simulink model "NOx_integrated_SIgnal_Builder"  (R2019a)
settings: Solver=FixedStepDiscrete  StartTime=0.0  StopTime=1500  FixedStep=0.1  RelTol=1e-3
undefined symbols (not defined in the file or in its folder): sigbuilder_block
settings Model: Creator=Kore  LastModifiedBy=admin
settings OptimizationCC: DefaultParameterBehavior=Inlined  EnhancedBackFolding=on  PassReuseOutputArgsAs=Individual arguments  OptimizeBlockOrder=speed  DifferentSizesBufferReuse=on  OptimizationCustomize=off
settings DebuggingCC: ParameterTunabilityLossMsg=error
settings SFSimCC: MATLABDynamicMemAlloc=off
settings RTWCC: SystemTargetFile=ert.tlc  GenCodeOnly=on  TemplateMakefile=ert_default_tmf  GenerateReport=on  IncludeHyperlinkInReport=on  LaunchReport=on  GenerateTraceInfo=on  GenerateTraceReport=on  GenerateTraceReportSl=on  GenerateTraceReportSf=on  GenerateTraceReportEml=on
settings CodeAppCC: ForceParamTrailComments=on  IgnoreCustomStorageClasses=off  OperatorAnnotations=on  SimulinkDataObjDesc=on  SFDataObjDesc=on  InsertBlockDesc=on
settings ERTTargetCC: TargetLangStandard=C99 (ISO)  GenerateSampleERTMain=on  InlinedParameterPlacement=NonHierarchical  ERTCustomFileTemplate=example_file_process.tlc
settings ConfigComp: CovEnable=on  RecordCoverage=on  CovMetricSettings=dcmwe  CovModelRefEnable=on

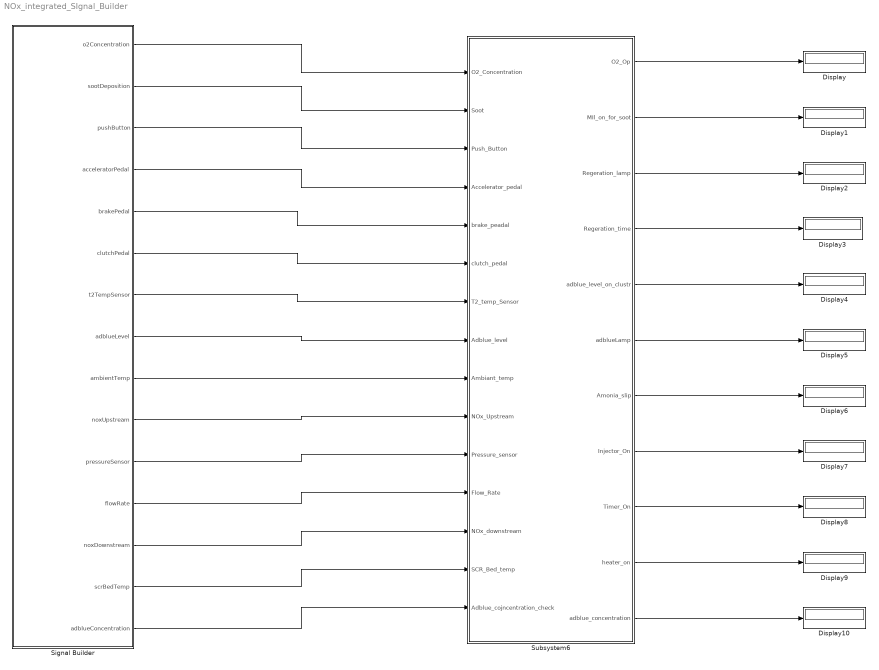
== system NOx_integrated_SIgnal_Builder ==
  Display{,1..10} (11 alike) : Display
  Signal Builder : Subsystem  Tag=STV Subsys  LoadFcn=sigbuilder_block('load');  StartFcn=sigbuilder_block('start');  StopFcn=sigbuilder_block('stop');  ClipboardFcn=sigbuilder_block('clipboard');  mask(Sigbuilder block){tuvar=[0:10]}
      mask help: Simulink:masks:SigbuilderBlock_MD
      mask init:
      | if ~strcmp(get_param(bdroot(gcbh),'SimulationStatus'),'stopped') tuvar = sigbuilder_block('maskInit'); end
      settings: CopyFcn=sigbuilder_block('copy');  DeleteFcn=sigbuilder_block('delete');  ModelCloseFcn=sigbuilder_block('modelClose');  PreSaveFcn=sigbuilder_block('preSave');  PauseFcn=sigbuilder_block('pause');  ContinueFcn=sigbuilder_block('continue');  NameChangeFcn=sigbuilder_block('namechange');  OpenFcn=sigbuilder_block('open',[437.6 30.75 550.4 481.5 ]);  CloseFcn=sigbuilder_block('close');
      mask Display: plot(0, 0, 100, 100,[2, 2, 32, 32, 2], [68, 8, 8, 68, 68],[32, 2], [38, 38], [32, 19, 2],[53, 60, 44], [32, 17, 17, 2],[16, 16, 31, 31]);txt = getActiveGroup(gcbh);text(2, 100, txt,'verticalAlignment', 'top');
  Subsystem6 : Subsystem
  wires:
  Subsystem6/2(MIl_on_for_soot) -> Display1/1
  Subsystem6/8(Injector_On) -> Display7/1
  Subsystem6/11(adblue_concentration) -> Display10/1
  Subsystem6/9(Timer_On) -> Display8/1
  Subsystem6/5(adblue_level_on_clustr) -> Display4/1
  Subsystem6/1(O2_Op) -> Display/1
  Subsystem6/10(heater_on) -> Display9/1
  Subsystem6/7(Amonia_slip) -> Display6/1
  Subsystem6/3(Regeration_lamp) -> Display2/1
  Subsystem6/4(Regeration_time) -> Display3/1
  Subsystem6/6(adblueLamp) -> Display5/1
  Signal Builder/1(o2Concentration) -> Subsystem6/1(O2_Concentration)
  Signal Builder/2(sootDeposition) -> Subsystem6/2(Soot)
  Signal Builder/3(pushButton) -> Subsystem6/3(Push_Button)
  Signal Builder/4(acceleratorPedal) -> Subsystem6/4(Accelerator_pedal)
  Signal Builder/5(brakePedal) -> Subsystem6/5(brake_peadal)
  Signal Builder/6(clutchPedal) -> Subsystem6/6(clutch_pedal)
  Signal Builder/7(t2TempSensor) -> Subsystem6/7(T2_temp_Sensor)
  Signal Builder/8(adblueLevel) -> Subsystem6/8(Adblue_level)
  Signal Builder/9(ambientTemp) -> Subsystem6/9(Ambiant_temp)
  Signal Builder/10(noxUpstream) -> Subsystem6/10(NOx_Upstream)
  Signal Builder/11(pressureSensor) -> Subsystem6/11(Pressure_sensor)
  Signal Builder/12(flowRate) -> Subsystem6/12(Flow_Rate)
  Signal Builder/13(noxDownstream) -> Subsystem6/13(NOx_downstream)
  Signal Builder/14(scrBedTemp) -> Subsystem6/14(SCR_Bed_temp)
  Signal Builder/15(adblueConcentration) -> Subsystem6/15(Adblue_cojncentration_check)

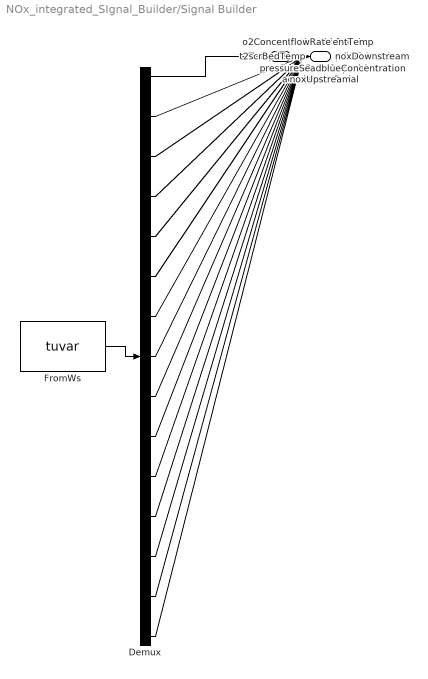
== system NOx_integrated_SIgnal_Builder/Signal Builder ==
  Demux : Demux  Tag=STV Demux  Outputs=15
  FromWs : FromWorkspace  Tag=STV FromWs  VariableName=tuvar  SampleTime=0
      SigBuilderData=|
      | common.afterFinalStr = 'Extrapolate'
      | common.sampleTime = 0
      | dataSet.timeRange = [0.1 77.4]
      | dataSet.name = 'Sheet1'
      | sbobj.Name = 'Signal Builder'
      | sbobj.Groups.Name = 'Sheet1'
      | sbobj.Groups.Signals(1).Name = 'o2Concentration'
      | sbobj.Groups.Signals(1).XData = [0.1 0.2 0.3 0.4 0.5 0.6 0.7 0.8 0.9 1 1.1 1.2 ... (774 elements, 1x774)]
      | sbobj.Groups.Signals(1).YData = [6.5 7 7.5 8 8.5 9 9.5 10 10.5 11 11.5 12 ... (774 elements, 1x774)]
      | sbobj.Groups.Signals(2).Name = 'sootDeposition'
      | sbobj.Groups.Signals(2).XData = [0.1 0.2 0.3 0.4 0.5 0.6 0.7 0.8 0.9 1 1.1 1.2 ... (774 elements, 1x774)]
      | sbobj.Groups.Signals(2).YData = [0.01 0.02 0.03 0.04 0.05 0.06 0.07 0.08 0.09 0.1 0.11 0.12 ... (774 elements, 1x774)]
      | sbobj.Groups.Signals(3).Name = 'pushButton'
      | sbobj.Groups.Signals(3).XData = [0.1 0.2 0.3 0.4 0.5 0.6 0.7 0.8 0.9 1 1.1 1.2 ... (774 elements, 1x774)]
      | sbobj.Groups.Signals(3).YData = [1 1 0 0 0 0 0 0 0 0 0 0 0 0 0 0 1 1 1 1 1 1 1 1 1 1 1 1 1 1 1 1 1 1 1 1 1 1 1 1 1 1 1 1 1 1 1 1 1 1 1 1 1 1 1 1 1 1 1 1 1 1 1 1 1 1 1 1 1 1 1 1 1 1 1 1 1 1 1 1 1 1 1 1 1 1 1 1 1 1 0 0 0 0 0 0 0 0 0 0 0 0 0 0 0 0 0 0 0 0 0 0 0 1 1 1 1 1 1 1 1 1 1 1 1 1 1 1 1 1 1 1 1 1 1 1 1 1 1 1 0 1 1 1 1 1 1 1 1 1 1 1 1 1 1 1 1 1 1 1 1 1 1 1 1 1 1 1 1 1 1 1 1 1 1 1 1 1 1 1 1 1 1 1 1 1 1 1 1 1 1 1 0 0 0 0 0 0 0 0 0 0 0 0 0 0 0 0 0 0 0 0 0 0 0 0 0 0 0 0 0 0 0 0 1 1 1 1 1 1 1 1 1 1 1 1 1 1 1 1 1 1 1 1 1 1 1 1 1 1 1 1 1 1 1 1 1 1 1 1 1 1 1 1 1 1 1 1 1 1 1 1 1 1 1 1 1 1 1 1 1 1 1 1 1 1 1 1 1 1 1 1 1 1 1 1 1 1 1 1 1 0 0 0 0 0 0 0 0 0 0 0 0 0 0 0 0 0 0 0 0 0 0 0 0 0 1 1 1 1 1 1 1 1 1 1 1 1 1 1 1 1 1 1 1 1 1 1 1 1 1 1 1 1 1 1 1 1 1 1 1 1 1 1 1 1 1 1 1 1 1 1 1 1 1 1 1 1 1 1 1 1 1 1 1 1 1 1 1 1 1 1 1 1 1 1 1 1 1 1 1 1 1 1 1 1 1 1 1 1 1 1 1 1 1 1 1 1 1 1 1 1 1 1 1 1 1 1 1 1 1 1 1 1 1 1 1 1 1 1 1 1 1 1 1 1 1 1 1 1 1 1 1 1 1 1 1 1 1 1 1 1 1 1 1 1 1 1 1 1 1 1 1 1 1 1 1 1 1 1 1 1 1 1 1 1 1 1 1 1 1 1 1 1 1 1 1 1 1 1 1 1 1 1 1 1 1 1 1 1 1 1 1 1 1 1 1 1 1 1 1 1 1 1 1 1 1 1 1 1 1 1 1 1 1 1 1 1 1 1 1 1 1 1 1 1 1 1 1 1 1 1 1 1 1 1 1 1 1 1 1 1 1 1 1 1 1 1 1 1 1 1 1 1 1 1 1 1 1 1 1 1 1 1 1 1 1 1 1 1 1 1 1 1 1 1 1 1 1 1 1 1 1 1 1 1 1 1 1 1 1 1 1 1 1 1 1 1 1 1 1 1 1 1 1 1 1 1 1 1 1 1 1 1 1 1 1 1 1 1 1 1 1 1 1 1 1 1 1 1 1 1 1 1 1 1 1 1 1 1 1 1 1 1 1 1 1 1 1 1 1 1 1 1 1 1 1 1 1 1 1 1 1 1 1 1 1 1 1 1 1 1 1 1 1 1 1 1 1 1 1 1 1 1 1 1 1 1 1 1 1 1 1 1 1 1 1 1 1 1 1 1 1 1 1 1 1 1 1 1 1 1 1 1 1 1 1 1 1 1 1 1 1 1 1 1 0 0 0 0 0 0 0 0 1 1 1 1 1 1 1 1 1 0 0 0 0 0 0 0 0 0 1 1]
      | sbobj.Groups.Signals(4).Name = 'acceleratorPedal'
      | sbobj.Groups.Signals(4).XData = [0.1 0.2 0.3 0.4 0.5 0.6 0.7 0.8 0.9 1 1.1 1.2 ... (774 elements, 1x774)]
      | sbobj.Groups.Signals(4).YData = [0 0 0 0 0 0 0 0 0 0 0 0 0 0 0 0 0 0 0 0 0 0 0 0 0 0 0 0 1 1 1 1 1 1 1 1 1 1 1 1 1 1 1 1 1 1 1 1 1 1 1 1 1 0 0 0 0 0 0 0 0 0 0 0 0 0 0 0 0 0 0 0 0 0 0 0 0 0 0 0 0 0 0 0 0 0 0 0 0 0 0 0 0 0 0 0 0 0 0 0 0 0 0 0 0 0 0 0 0 0 0 0 0 0 0 0 0 0 0 0 0 0 0 0 0 0 0 0 0 0 0 0 0 0 0 0 0 0 0 0 0 0 0 0 0 1 0 0 0 0 0 0 1 0 0 0 0 0 1 1 0 0 0 0 0 1 0 0 0 0 0 0 0 0 0 0 0 1 0 0 0 0 0 1 0 0 1 0 0 0 0 0 0 0 0 0 0 0 0 0 0 0 0 0 0 0 0 0 0 0 0 0 0 0 0 0 0 0 0 0 0 0 0 0 0 0 0 0 0 0 0 0 0 0 0 0 0 0 0 0 0 0 0 0 0 0 0 0 0 0 0 0 0 0 0 0 0 0 0 0 0 0 0 0 0 0 0 0 0 0 0 0 0 0 0 0 0 0 0 0 0 0 0 0 0 0 0 0 0 0 0 0 0 0 0 0 0 0 0 0 0 1 1 1 1 1 1 1 1 1 1 1 1 1 1 1 1 1 1 1 1 1 1 1 1 1 0 0 0 0 0 0 0 0 0 0 0 0 0 0 0 0 0 0 0 0 0 0 0 0 0 0 0 0 0 0 0 0 0 0 0 0 0 0 0 0 0 0 0 0 0 0 0 0 0 0 0 0 0 0 0 0 0 0 0 0 0 0 0 0 0 0 0 0 0 0 0 0 0 0 0 0 0 0 0 0 0 0 0 0 0 0 0 0 0 0 0 0 0 0 0 0 0 0 0 0 0 0 0 0 0 0 0 0 0 0 0 0 0 0 0 0 0 0 0 0 0 0 0 0 0 0 0 0 0 0 0 0 0 0 0 0 0 0 0 0 0 0 0 0 0 0 0 0 0 0 0 0 0 0 0 0 0 0 0 0 0 0 0 0 0 0 0 0 0 0 0 0 0 0 0 0 0 0 0 0 0 0 0 0 0 0 0 0 0 0 0 0 0 0 0 0 0 0 0 0 0 0 0 0 0 0 0 0 0 0 0 0 0 0 0 0 0 0 0 1 0 0 0 0 0 0 1 0 0 0 0 0 1 1 0 0 0 0 0 1 0 0 0 0 0 0 0 0 0 0 0 1 0 0 0 0 0 1 0 0 1 0 0 0 0 0 0 0 0 0 0 0 0 0 0 0 0 0 0 0 0 0 0 0 0 0 0 0 0 0 0 0 0 0 0 0 0 0 0 0 0 0 0 0 0 0 0 0 0 0 0 0 0 0 0 0 0 0 0 0 0 0 0 0 0 0 0 0 0 0 0 0 0 0 0 0 0 0 0 0 0 0 0 0 0 0 0 0 0 0 0 0 0 0 0 0 0 0 0 0 0 0 0 0 0 0 0 0 0 0 0 0 0 0 0 0 0 0 0 0 0 0 0 0 0 0 0 0 0 0 0 1 1 0 1 0 0 0 1 1 1 1 1 1 1 1 0 0 0 1 1 1 1 0 0 0 0 1 1 1 0 0 0 0 1 1 1 0 0 0 0 1 1 1 0 0 0 0 0 0 0 0 1 1 1 0 0 0]
      | sbobj.Groups.Signals(5).Name = 'brakePedal'
      | sbobj.Groups.Signals(5).XData = [0.1 0.2 0.3 0.4 0.5 0.6 0.7 0.8 0.9 1 1.1 1.2 ... (774 elements, 1x774)]
      | sbobj.Groups.Signals(5).YData = [0 0 0 0 0 0 0 0 0 0 0 0 0 0 0 0 0 0 0 0 0 0 0 0 0 0 0 0 1 1 1 1 1 1 1 1 1 1 1 1 1 1 1 1 1 1 1 1 1 1 1 1 1 0 0 0 0 0 0 0 0 0 0 0 0 0 0 0 0 0 0 0 0 0 0 0 0 0 0 0 0 0 0 0 0 0 0 0 0 0 0 0 0 0 0 0 0 0 0 0 0 0 0 0 0 0 0 0 0 0 0 0 0 0 0 0 0 0 0 0 0 0 0 0 0 0 0 0 0 0 0 0 0 0 0 0 0 0 0 0 0 0 0 0 0 0 1 0 0 0 0 0 0 1 0 0 0 1 0 0 1 0 0 1 0 0 0 0 0 1 0 1 0 1 0 0 0 0 0 0 0 0 0 0 0 0 0 0 0 0 0 0 0 0 0 0 0 0 0 0 0 0 0 0 0 0 0 0 0 0 0 0 0 0 0 0 0 0 0 0 0 0 0 0 0 0 0 0 0 0 0 0 0 0 0 0 0 0 0 0 0 0 0 0 0 0 0 0 0 0 0 0 0 0 0 0 0 0 0 0 0 0 0 0 0 0 0 0 0 0 0 0 0 0 0 0 0 0 0 0 0 0 0 0 0 0 0 0 0 0 0 0 0 0 0 0 0 0 0 0 0 1 1 1 1 1 1 1 1 1 1 1 1 1 1 1 1 1 1 1 1 1 1 1 1 1 0 0 0 0 0 0 0 0 0 0 0 0 0 0 0 0 0 0 0 0 0 0 0 0 0 0 0 0 0 0 0 0 0 0 0 0 0 0 0 0 0 0 0 0 0 0 0 0 0 0 0 0 0 0 0 0 0 0 0 0 0 0 0 0 0 0 0 0 0 0 0 0 0 0 0 0 0 0 0 0 0 0 0 0 0 0 0 0 0 0 0 0 0 0 0 0 0 0 0 0 0 0 0 0 0 0 0 0 0 0 0 0 0 0 0 0 0 0 0 0 0 0 0 0 0 0 0 0 0 0 0 0 0 0 0 0 0 0 0 0 0 0 0 0 0 0 0 0 0 0 0 0 0 0 0 0 0 0 0 0 0 0 0 0 0 0 0 0 0 0 0 0 0 0 0 0 0 0 0 0 0 0 0 0 0 0 0 0 0 0 0 0 0 0 0 0 0 0 0 0 0 0 0 0 0 0 0 0 0 0 0 0 0 0 0 0 0 0 0 0 1 0 0 0 0 0 0 1 0 0 0 1 0 0 1 0 0 1 0 0 0 0 0 1 0 1 0 1 0 0 0 0 0 0 0 0 0 0 0 0 0 0 0 0 0 0 0 0 0 0 0 0 0 0 0 0 0 0 0 0 0 0 0 0 0 0 0 0 0 0 0 0 0 0 0 0 0 0 0 0 0 0 0 0 0 0 0 0 0 0 0 0 0 0 0 0 0 0 0 0 0 0 0 0 0 0 0 0 0 0 0 0 0 0 0 0 0 0 0 0 0 0 0 0 0 0 0 0 0 0 0 0 0 0 0 0 0 0 0 0 0 0 0 0 0 0 0 0 0 0 0 0 0 0 0 0 0 0 0 0 0 0 0 0 0 0 0 0 0 0 0 1 1 0 1 0 0 1 1 1 1 1 1 1 1 1 0 0 0 1 1 1 1 0 0 0 0 1 1 1 0 0 0 0 1 1 1 0 0 0 0 1 1 1 0 0 0 0 0 0 0 0 1 1 1 0 0 0]
      | sbobj.Groups.Signals(6).Name = 'clutchPedal'
      | sbobj.Groups.Signals(6).XData = [0.1 0.2 0.3 0.4 0.5 0.6 0.7 0.8 0.9 1 1.1 1.2 ... (774 elements, 1x774)]
      | sbobj.Groups.Signals(6).YData = [0 0 0 0 0 0 0 0 0 0 0 0 0 0 0 0 0 0 0 0 0 0 0 0 0 0 0 0 1 1 1 1 1 1 1 1 1 1 1 1 1 1 1 1 1 1 1 1 1 1 1 1 1 0 0 0 0 0 0 0 0 0 0 0 0 0 0 0 0 0 0 0 0 0 0 0 0 0 0 0 0 0 0 0 0 0 0 0 0 0 0 0 0 0 0 0 0 0 0 0 0 0 0 0 0 0 0 0 0 0 0 0 0 0 0 0 0 0 0 0 0 0 0 0 0 0 0 0 0 0 0 0 0 0 0 0 0 0 0 0 0 0 0 0 0 0 0 1 0 0 0 0 0 0 1 0 0 0 1 0 0 0 0 0 1 0 0 0 0 0 0 0 0 0 0 1 0 0 1 0 0 0 0 0 1 0 0 0 0 0 0 0 0 0 0 0 0 0 0 0 0 0 0 0 0 0 0 0 0 0 0 0 0 0 0 0 0 0 0 0 0 0 0 0 0 0 0 0 0 0 0 0 0 0 0 0 0 0 0 0 0 0 0 0 0 0 0 0 0 0 0 0 0 0 0 0 0 0 0 0 0 0 0 0 0 0 0 0 0 0 0 0 0 0 0 0 0 0 0 0 0 0 0 0 0 0 0 0 0 0 0 0 0 0 0 0 0 0 0 0 0 1 1 1 1 1 1 1 1 1 1 1 1 1 1 1 1 1 1 1 1 1 1 1 1 1 0 0 0 0 0 0 0 0 0 0 0 0 0 0 0 0 0 0 0 0 0 0 0 0 0 0 0 0 0 0 0 0 0 0 0 0 0 0 0 0 0 0 0 0 0 0 0 0 0 0 0 0 0 0 0 0 0 0 0 0 0 0 0 0 0 0 0 0 0 0 0 0 0 0 0 0 0 0 0 0 0 0 0 0 0 0 0 0 0 0 0 0 0 0 0 0 0 0 0 0 0 0 0 0 0 0 0 0 0 0 0 0 0 0 0 0 0 0 0 0 0 0 0 0 0 0 0 0 0 0 0 0 0 0 0 0 0 0 0 0 0 0 0 0 0 0 0 0 0 0 0 0 0 0 0 0 0 0 0 0 0 0 0 0 0 0 0 0 0 0 0 0 0 0 0 0 0 0 0 0 0 0 0 0 0 0 0 0 0 0 0 0 0 0 0 0 0 0 0 0 0 0 0 0 0 0 0 0 0 0 0 0 0 0 0 0 0 0 0 0 0 1 0 0 0 0 0 0 1 0 0 0 1 0 0 0 0 0 1 0 0 0 0 0 0 0 0 0 0 1 0 0 1 0 0 0 0 0 1 0 0 0 0 0 0 0 0 0 0 0 0 0 0 0 0 0 0 0 0 0 0 0 0 0 0 0 0 0 0 0 0 0 0 0 0 0 0 0 0 0 0 0 0 0 0 0 0 0 0 0 0 0 0 0 0 0 0 0 0 0 0 0 0 0 0 0 0 0 0 0 0 0 0 0 0 0 0 0 0 0 0 0 0 0 0 0 0 0 0 0 0 0 0 0 0 0 0 0 0 0 0 0 0 0 0 0 0 0 0 0 0 0 0 0 0 0 0 0 0 0 0 0 0 0 0 0 0 0 0 0 0 1 1 0 1 0 0 0 1 1 1 1 1 1 1 1 0 0 0 1 1 1 1 0 0 0 0 1 1 1 0 0 0 0 1 1 1 0 0 0 0 1 1 1 0 0 0 0 0 0 0 0 1 1 1 0 0 0]
      | sbobj.Groups.Signals(7).Name = 't2TempSensor'
      | sbobj.Groups.Signals(7).XData = [0.1 0.2 0.3 0.4 0.5 0.6 0.7 0.8 0.9 1 1.1 1.2 ... (774 elements, 1x774)]
      | sbobj.Groups.Signals(7).YData = [310 320 330 340 350 360 370 380 390 400 410 420 ... (774 elements, 1x774)]
      | sbobj.Groups.Signals(8).Name = 'adblueLevel'
      | sbobj.Groups.Signals(8).XData = [0.1 0.2 0.3 0.4 0.5 0.6 0.7 0.8 0.9 1 1.1 1.2 ... (774 elements, 1x774)]
      | sbobj.Groups.Signals(8).YData = [1 2 3 4 5 6 7 8 9 10 11 12 ... (774 elements, 1x774)]
      | sbobj.Groups.Signals(9).Name = 'ambientTemp'
      | sbobj.Groups.Signals(9).XData = [0.1 0.2 0.3 0.4 0.5 0.6 0.7 0.8 0.9 1 1.1 1.2 ... (774 elements, 1x774)]
      | sbobj.Groups.Signals(9).YData = [0 1 2 3 4 5 6 7 8 9 10 11 ... (774 elements, 1x774)]
      | sbobj.Groups.Signals(10).Name = 'noxUpstream'
      | sbobj.Groups.Signals(10).XData = [0.1 0.2 0.3 0.4 0.5 0.6 0.7 0.8 0.9 1 1.1 1.2 ... (774 elements, 1x774)]
      | sbobj.Groups.Signals(10).YData = [10 70 77.6 80.4 86.4 99.6 108 117.6 127.2 136.8 149.3 158.3 ... (774 elements, 1x774)]
      | sbobj.Groups.Signals(11).Name = 'pressureSensor'
      | sbobj.Groups.Signals(11).XData = [0.1 0.2 0.3 0.4 0.5 0.6 0.7 0.8 0.9 1 1.1 1.2 ... (774 elements, 1x774)]
      | sbobj.Groups.Signals(11).YData = [5.8 5.8 5.8 5.8 5.8 5.8 5.8 5.8 5.8 5.8 5.8 5.8 ... (774 elements, 1x774)]
      | sbobj.Groups.Signals(12).Name = 'flowRate'
      | sbobj.Groups.Signals(12).XData = [0.1 0.2 0.3 0.4 0.5 0.6 0.7 0.8 0.9 1 1.1 1.2 ... (774 elements, 1x774)]
      | sbobj.Groups.Signals(12).YData = [3 3 3 3 3 4 4 4 4 4.8 4.8 4.8 ... (774 elements, 1x774)]
      | sbobj.Groups.Signals(13).Name = 'noxDownstream'
      | sbobj.Groups.Signals(13).XData = [0.1 0.2 0.3 0.4 0.5 0.6 0.7 0.8 0.9 1 1.1 1.2 ... (774 elements, 1x774)]
      | sbobj.Groups.Signals(13).YData = [15 15 15 14 14 14 14 15 15 15 15 17 ... (774 elements, 1x774)]
      | sbobj.Groups.Signals(14).Name = 'scrBedTemp'
      | sbobj.Groups.Signals(14).XData = [0.1 0.2 0.3 0.4 0.5 0.6 0.7 0.8 0.9 1 1.1 1.2 ... (774 elements, 1x774)]
      | sbobj.Groups.Signals(14).YData = [1 10 20 30 40 50 60 70 80 90 100 110 ... (774 elements, 1x774)]
      | sbobj.Groups.Signals(15).Name = 'adblueConcentration'
      | sbobj.Groups.Signals(15).XData = [0.1 0.2 0.3 0.4 0.5 0.6 0.7 0.8 0.9 1 1.1 1.2 ... (774 elements, 1x774)]
      | sbobj.Groups.Signals(15).YData = [31.5 31.6 31.7 31.8 31.9 32 32.1 32.2 32.3 32.4 32.5 32.6 ... (774 elements, 1x774)]
      | sbobj.Groups.TimeRange = [0.1 73.9]
  o2Concentration : Outport  Tag=STV Outport
  sootDeposition : Outport  Tag=STV Outport  Port=2
  pushButton : Outport  Tag=STV Outport  Port=3
  acceleratorPedal : Outport  Tag=STV Outport  Port=4
  brakePedal : Outport  Tag=STV Outport  Port=5
  clutchPedal : Outport  Tag=STV Outport  Port=6
  t2TempSensor : Outport  Tag=STV Outport  Port=7
  adblueLevel : Outport  Tag=STV Outport  Port=8
  ambientTemp : Outport  Tag=STV Outport  Port=9
  noxUpstream : Outport  Tag=STV Outport  Port=10
  pressureSensor : Outport  Tag=STV Outport  Port=11
  flowRate : Outport  Tag=STV Outport  Port=12
  noxDownstream : Outport  Tag=STV Outport  Port=13
  scrBedTemp : Outport  Tag=STV Outport  Port=14
  adblueConcentration : Outport  Tag=STV Outport  Port=15
  wires:
  Demux/1 -> o2Concentration/1
  FromWs/1 -> Demux/1
  Demux/2 -> sootDeposition/1
  Demux/3 -> pushButton/1
  Demux/4 -> acceleratorPedal/1
  Demux/5 -> brakePedal/1
  Demux/6 -> clutchPedal/1
  Demux/7 -> t2TempSensor/1
  Demux/8 -> adblueLevel/1
  Demux/9 -> ambientTemp/1
  Demux/10 -> noxUpstream/1
  Demux/11 -> pressureSensor/1
  Demux/12 -> flowRate/1
  Demux/13 -> noxDownstream/1
  Demux/14 -> scrBedTemp/1
  Demux/15 -> adblueConcentration/1

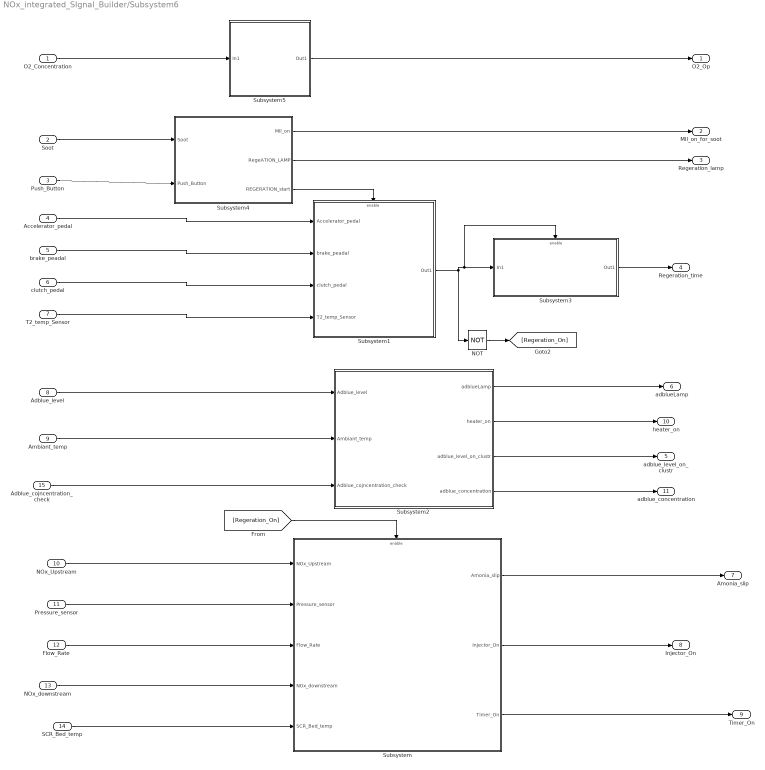
== system NOx_integrated_SIgnal_Builder/Subsystem6 ==
  O2_Concentration : Inport
  Soot : Inport  Port=2
  Push_Button : Inport  Port=3
  Accelerator_pedal : Inport  Port=4
  brake_peadal : Inport  Port=5
  clutch_pedal : Inport  Port=6
  T2_temp_Sensor : Inport  Port=7
  Adblue_level : Inport  Port=8
  Ambiant_temp : Inport  Port=9
  NOx_Upstream : Inport  Port=10
  Pressure_sensor : Inport  Port=11
  Flow_Rate : Inport  Port=12
  NOx_downstream : Inport  Port=13
  SCR_Bed_temp : Inport  Port=14
  Adblue_cojncentration_check : Inport  Port=15
  NOT : Logic  Operator=NOT  IconShape=distinctive  AllPortsSameDT=off  OutDataTypeStr=boolean
  Subsystem : Subsystem
  Subsystem1 : Subsystem
  Subsystem2 : Subsystem
  Subsystem3 : Subsystem
  Subsystem4 : Subsystem
  Subsystem5 : Subsystem
  O2_Op : Outport
  MIl_on_for_soot : Outport  Port=2
  Regeration_lamp : Outport  Port=3
  Regeration_time : Outport  Port=4
  adblue_level_on_clustr : Outport  Port=5
  adblueLamp : Outport  Port=6
  Amonia_slip : Outport  Port=7
  Injector_On : Outport  Port=8
  Timer_On : Outport  Port=9
  heater_on : Outport  Port=10
  adblue_concentration : Outport  Port=11
  wires:
  T2_temp_Sensor/1 -> Subsystem1/4(T2_temp_Sensor)
  NOT/1 -> [Regeration_On]
  Subsystem/3(Timer_On) -> Timer_On/1
  Subsystem1/1(Out1) -> Subsystem3/Enable, Subsystem3/1(In1), NOT/1
  Push_Button/1 -> Subsystem4/2(Push_Button)
  Subsystem4/3(REGERATION_start) -> Subsystem1/Enable
  Subsystem/1(Amonia_slip) -> Amonia_slip/1
  NOx_Upstream/1 -> Subsystem/1(NOx_Upstream)
  Subsystem5/1(Out1) -> O2_Op/1
  Subsystem4/2(RegeATION_LAMP) -> Regeration_lamp/1
  [Regeration_On] -> Subsystem/Enable
  Adblue_level/1 -> Subsystem2/1(Adblue_level)
  O2_Concentration/1 -> Subsystem5/1(In1)
  clutch_pedal/1 -> Subsystem1/3(clutch_pedal)
  Accelerator_pedal/1 -> Subsystem1/1(Accelerator_pedal)
  Flow_Rate/1 -> Subsystem/3(Flow_Rate)
  Soot/1 -> Subsystem4/1(Soot)
  Pressure_sensor/1 -> Subsystem/2(Pressure_sensor)
  Subsystem/2(Injector_On) -> Injector_On/1
  NOx_downstream/1 -> Subsystem/4(NOx_downstream)
  SCR_Bed_temp/1 -> Subsystem/5(SCR_Bed_temp)
  Subsystem4/1(MIl_on) -> MIl_on_for_soot/1
  brake_peadal/1 -> Subsystem1/2("brake_peadal ")
  Ambiant_temp/1 -> Subsystem2/2(Ambiant_temp)
  Subsystem2/1(adblueLamp) -> adblueLamp/1
  Subsystem2/3(adblue_level_on_clustr) -> adblue_level_on_clustr/1
  Subsystem2/2(heater_on) -> heater_on/1
  Adblue_cojncentration_check/1 -> Subsystem2/3(Adblue_cojncentration_check)
  Subsystem2/4(adblue_concentration) -> adblue_concentration/1
  Subsystem3/1(Out1) -> Regeration_time/1

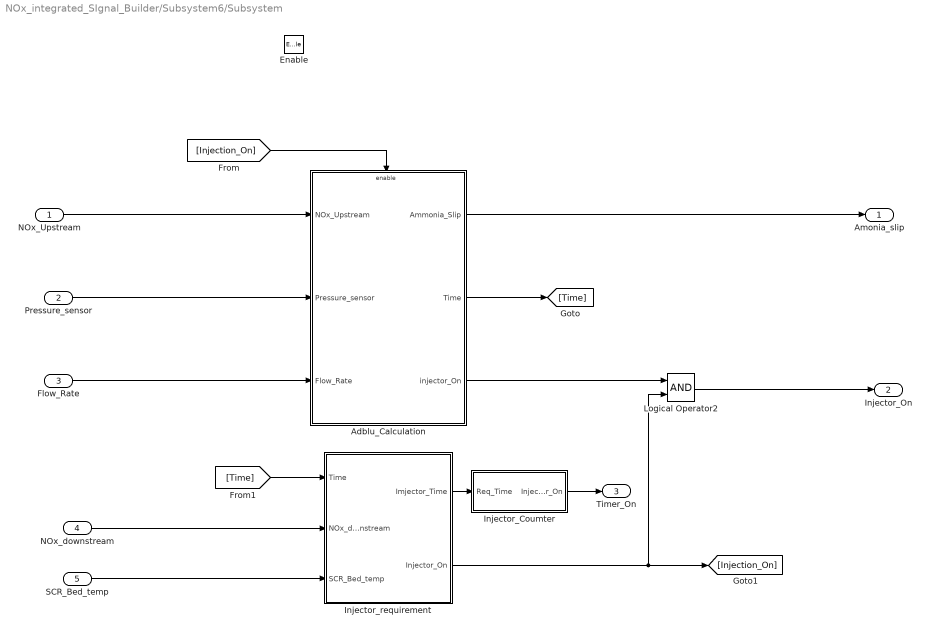
== system NOx_integrated_SIgnal_Builder/Subsystem6/Subsystem ==
  NOx_Upstream : Inport
  Pressure_sensor : Inport  Port=2
  Flow_Rate : Inport  Port=3
  NOx_downstream : Inport  Port=4
  SCR_Bed_temp : Inport  Port=5
  Enable : EnablePort
  Adblu_Calculation : Subsystem
  Injector_Coumter : Subsystem
  Injector_requirement : Subsystem
  Logical Operator2 : Logic  AllPortsSameDT=off  OutDataTypeStr=boolean
  Amonia_slip : Outport
  Injector_On : Outport  Port=2
  Timer_On : Outport  Port=3
  wires:
  Adblu_Calculation/2(Time) -> [Time]
  [Time] -> Injector_requirement/1(Time)
  Injector_Coumter/1(Injector_On) -> Timer_On/1
  Logical Operator2/1 -> Injector_On/1
  Injector_requirement/2(Injector_On) -> Logical Operator2/2, [Injection_On]
  Injector_requirement/1(Imjector_Time) -> Injector_Coumter/1(Req_Time)
  Adblu_Calculation/3(injector_On) -> Logical Operator2/1
  [Injection_On] -> Adblu_Calculation/Enable
  Adblu_Calculation/1(Ammonia_Slip) -> Amonia_slip/1
  NOx_downstream/1 -> Injector_requirement/2(NOx_downstream)
  NOx_Upstream/1 -> Adblu_Calculation/1(NOx_Upstream)
  SCR_Bed_temp/1 -> Injector_requirement/3(SCR_Bed_temp)
  Pressure_sensor/1 -> Adblu_Calculation/2(Pressure_sensor)
  Flow_Rate/1 -> Adblu_Calculation/3(Flow_Rate)

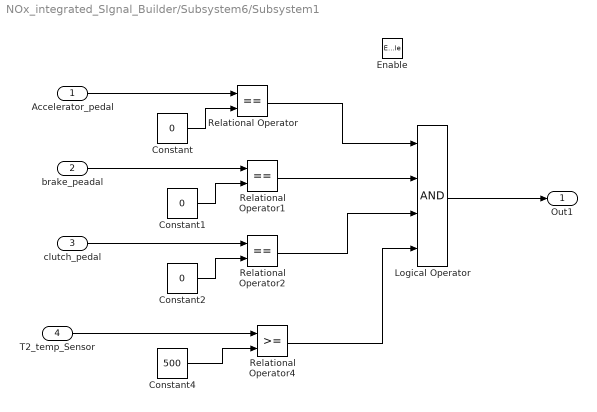
== system NOx_integrated_SIgnal_Builder/Subsystem6/Subsystem1 ==
  Accelerator_pedal : Inport
  "brake_peadal " : Inport  Port=2
  clutch_pedal : Inport  Port=3
  T2_temp_Sensor : Inport  Port=4
  Enable : EnablePort  StatesWhenEnabling=reset
  Constant : Constant  Value=0
  Constant1 : Constant  Value=0
  Constant2 : Constant  Value=0
  Constant4 : Constant  Value=500
  Logical Operator : Logic  Inputs=4  AllPortsSameDT=off  OutDataTypeStr=boolean
  Relational Operator : RelationalOperator  Operator===  OutDataTypeStr=boolean  RndMeth=Simplest
  Relational Operator1 : RelationalOperator  Operator===  OutDataTypeStr=boolean  RndMeth=Simplest
  Relational Operator2 : RelationalOperator  Operator===  OutDataTypeStr=boolean  RndMeth=Simplest
  Relational Operator4 : RelationalOperator  OutDataTypeStr=boolean  RndMeth=Simplest
  Out1 : Outport
  wires:
  Constant/1 -> Relational Operator/2
  Accelerator_pedal/1 -> Relational Operator/1
  "brake_peadal "/1 -> Relational Operator1/1
  Constant1/1 -> Relational Operator1/2
  Constant2/1 -> Relational Operator2/2
  clutch_pedal/1 -> Relational Operator2/1
  Relational Operator/1 -> Logical Operator/1
  Relational Operator1/1 -> Logical Operator/2
  Relational Operator2/1 -> Logical Operator/3
  T2_temp_Sensor/1 -> Relational Operator4/1
  Constant4/1 -> Relational Operator4/2
  Logical Operator/1 -> Out1/1
  Relational Operator4/1 -> Logical Operator/4

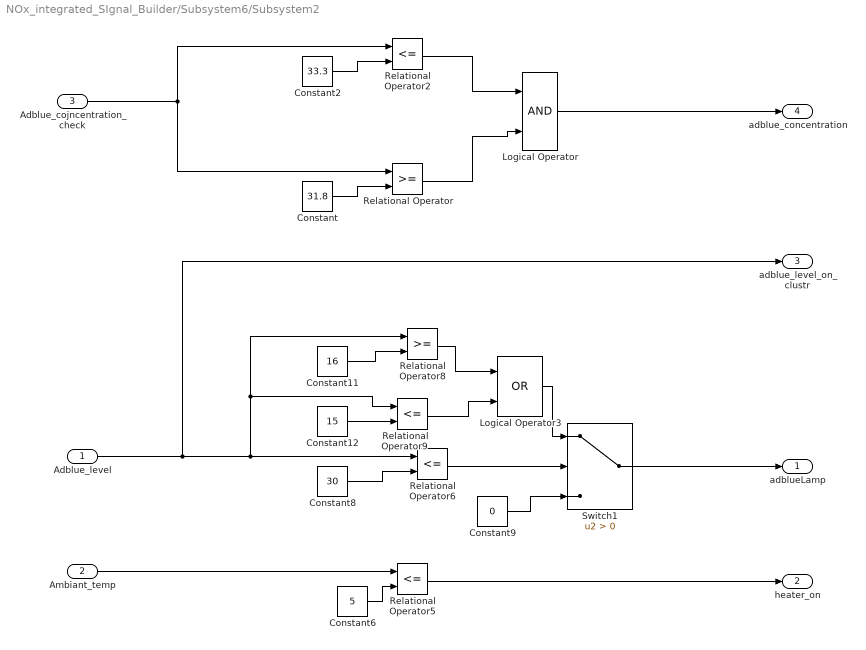
== system NOx_integrated_SIgnal_Builder/Subsystem6/Subsystem2 ==
  Adblue_level : Inport
  Ambiant_temp : Inport  Port=2
  Adblue_cojncentration_check : Inport  Port=3
  Constant : Constant  Value=31.8
  Constant11 : Constant  Value=16
  Constant12 : Constant  Value=15
  Constant2 : Constant  Value=33.3
  Constant6 : Constant  Value=5  OutDataTypeStr=int8
  Constant8 : Constant  Value=30
  Constant9 : Constant  Value=0
  Logical Operator : Logic  AllPortsSameDT=off  OutDataTypeStr=boolean
  Logical Operator3 : Logic  Operator=OR  AllPortsSameDT=off  OutDataTypeStr=boolean
  Relational Operator : RelationalOperator  OutDataTypeStr=boolean  RndMeth=Simplest
  Relational Operator{2,5..6,9} (4 alike) : RelationalOperator  Operator=<=  OutDataTypeStr=boolean  RndMeth=Simplest
  Relational Operator8 : RelationalOperator  OutDataTypeStr=boolean  RndMeth=Simplest
  Switch1 : Switch  Criteria=u2 > Threshold
  adblueLamp : Outport
  heater_on : Outport  Port=2
  adblue_level_on_clustr : Outport  Port=3
  adblue_concentration : Outport  Port=4
  wires:
  Logical Operator3/1 -> Switch1/1
  Constant9/1 -> Switch1/3
  Adblue_level/1 -> adblue_level_on_clustr/1, Relational Operator6/1, Relational Operator9/1, Relational Operator8/1
  Constant11/1 -> Relational Operator8/2
  Constant8/1 -> Relational Operator6/2
  Constant12/1 -> Relational Operator9/2
  Relational Operator6/1 -> Switch1/2
  Constant6/1 -> Relational Operator5/2
  Relational Operator5/1 -> heater_on/1
  Switch1/1 -> adblueLamp/1
  Ambiant_temp/1 -> Relational Operator5/1
  Constant/1 -> Relational Operator/2
  Adblue_cojncentration_check/1 -> Relational Operator/1, Relational Operator2/1
  Constant2/1 -> Relational Operator2/2
  Relational Operator2/1 -> Logical Operator/1
  Relational Operator/1 -> Logical Operator/2
  Logical Operator/1 -> adblue_concentration/1
  Relational Operator8/1 -> Logical Operator3/1
  Relational Operator9/1 -> Logical Operator3/2

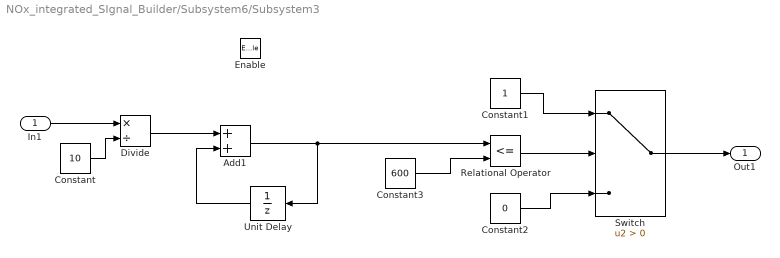
== system NOx_integrated_SIgnal_Builder/Subsystem6/Subsystem3 ==
  In1 : Inport
  Enable : EnablePort  StatesWhenEnabling=reset
  Add1 : Sum  OutDataTypeStr=double  RndMeth=Round
  Constant : Constant  Value=10
  Constant1 : Constant
  Constant2 : Constant  Value=0
  Constant3 : Constant  Value=600
  Divide : Product  Inputs=*/
  Relational Operator : RelationalOperator  Operator=<=  OutDataTypeStr=boolean  RndMeth=Simplest
  Switch : Switch  Criteria=u2 > Threshold
  Unit Delay : UnitDelay  InitialCondition=0.1  SampleTime=-1  HasFrameUpgradeWarning=on
  Out1 : Outport
  wires:
  Unit Delay/1 -> Add1/2
  In1/1 -> Divide/1
  Divide/1 -> Add1/1
  Constant/1 -> Divide/2
  Relational Operator/1 -> Switch/2
  Add1/1 -> Unit Delay/1, Relational Operator/1
  Constant2/1 -> Switch/3
  Constant1/1 -> Switch/1
  Constant3/1 -> Relational Operator/2
  Switch/1 -> Out1/1

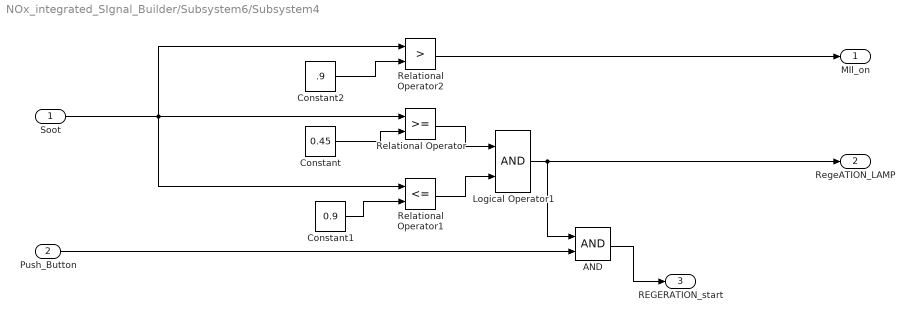
== system NOx_integrated_SIgnal_Builder/Subsystem6/Subsystem4 ==
  Soot : Inport
  Push_Button : Inport  Port=2
  AND : Logic  AllPortsSameDT=off  OutDataTypeStr=boolean
  Constant : Constant  Value=0.45
  Constant1 : Constant  Value=0.9
  Constant2 : Constant  Value=.9
  Logical Operator1 : Logic  AllPortsSameDT=off  OutDataTypeStr=boolean
  Relational Operator : RelationalOperator  OutDataTypeStr=boolean  RndMeth=Simplest
  Relational Operator1 : RelationalOperator  Operator=<=  OutDataTypeStr=boolean  RndMeth=Simplest
  Relational Operator2 : RelationalOperator  Operator=>  OutDataTypeStr=boolean  RndMeth=Simplest
  MIl_on : Outport
  RegeATION_LAMP : Outport  Port=2
  REGERATION_start : Outport  Port=3
  wires:
  Soot/1 -> Relational Operator1/1, Relational Operator2/1, Relational Operator/1
  AND/1 -> REGERATION_start/1
  Logical Operator1/1 -> AND/1, RegeATION_LAMP/1
  Constant2/1 -> Relational Operator2/2
  Push_Button/1 -> AND/2
  Constant1/1 -> Relational Operator1/2
  Constant/1 -> Relational Operator/2
  Relational Operator1/1 -> Logical Operator1/2
  Relational Operator2/1 -> MIl_on/1
  Relational Operator/1 -> Logical Operator1/1

== system NOx_integrated_SIgnal_Builder/Subsystem6/Subsystem5 ==
  In1 : Inport
  AND : Logic  AllPortsSameDT=off  OutDataTypeStr=boolean
  Constant3 : Constant  Value=8
  Constant4 : Constant  Value=14.5
  Relational Operator3 : RelationalOperator  OutDataTypeStr=boolean  RndMeth=Simplest
  Relational Operator4 : RelationalOperator  Operator=<=  OutDataTypeStr=boolean  RndMeth=Simplest
  Out1 : Outport
  wires:
  Constant3/1 -> Relational Operator3/2
  Relational Operator3/1 -> AND/1
  AND/1 -> Out1/1
  In1/1 -> Relational Operator4/1, Relational Operator3/1
  Constant4/1 -> Relational Operator4/2
  Relational Operator4/1 -> AND/2

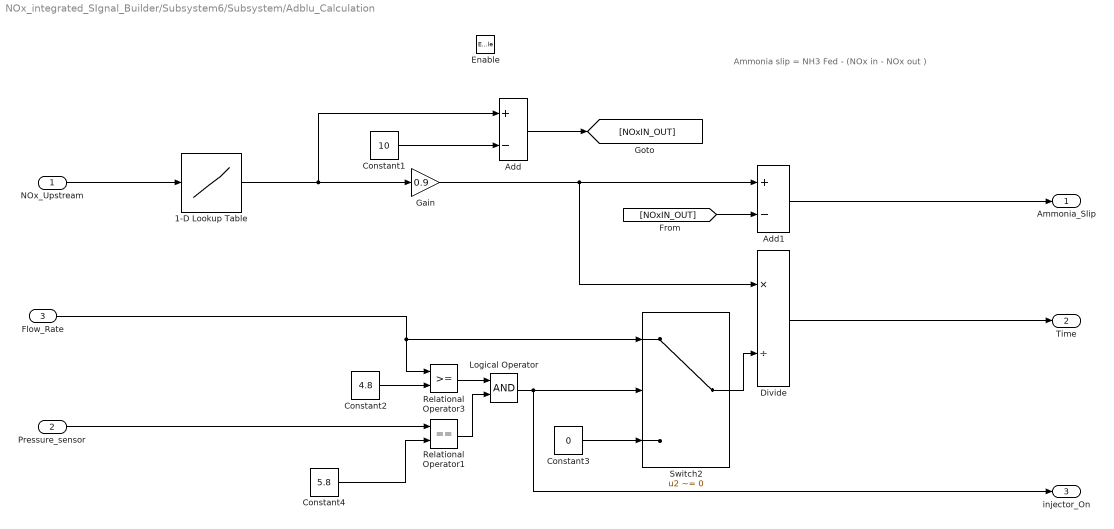
== system NOx_integrated_SIgnal_Builder/Subsystem6/Subsystem/Adblu_Calculation ==
  note: Ammonia slip = NH3 Fed - (NOx in - NOx out )
  NOx_Upstream : Inport
  Pressure_sensor : Inport  Port=2
  Flow_Rate : Inport  Port=3
  Enable : EnablePort  StatesWhenEnabling=reset
  1-D Lookup Table : Lookup_n-D  NumberOfTableDimensions=1  BreakpointsForDimension1=|  BreakpointsForDimension1DataTypeStr=double  Table=|  TableDataTypeStr=double  IntermediateResultsDataTypeStr=double  InternalRulePriority=Speed  OutDataTypeStr=double  RndMeth=Simplest  FractionDataTypeStr=double  InputSameDT=on
      BreakpointsForDimension1=|
      | [10
      | 70
      | 77.6
      | 80.4
      | 86.4
      | 99.6
      | 108
      | 117.6
      | 127.2
      | 136.8
      | 149.3
      | 158.3
      | 163.3
      | 168.3
      | 175.3
      | 181.5
      | 187.7
      | 193.9
      | 200.1
      | 206.3
      | 212.85
      | 223.5
      | 233.15
      | 242.8
      | 255.45
      | 264.9
      | 275.35
      | 285.8
      | 296.25
      | 306.7
      | 317.15
      | 327.6
      | 338.05
      | 348.5
      | 358.95
      | 369.4
      | 379.85
      | 390.3
      | 400.75
      | 411.2
      | 421.65
      | 432.1
      | 442.55
      | 453
      | 463.45
      | 473.9
      | 484.35
      | 494.8
      | 505.25
      | 515.7
      | 526.15
      | 536.6
      | 547.05
      | 557.5
      | 567.95
      | 578.4
      | 588.85
      | 599.3
      | 609.75
      | 620.2
      | 630.65
      | 641.1
      | 651.55
      | 662
      | 672.45
      | 682.9
      | 693.35
      | 703.8
      | ]
      Table=|
      | [10
      | 70
      | 77.6
      | 80.4
      | 86.4
      | 99.6
      | 108
      | 117.6
      | 127.2
      | 136.8
      | 149.3
      | 158.3
      | 163.3
      | 168.3
      | 175.3
      | 181.5
      | 187.7
      | 193.9
      | 200.1
      | 206.3
      | 212.85
      | 223.5
      | 233.15
      | 242.8
      | 255.45
      | 264.9
      | 275.35
      | 285.8
      | 296.25
      | 306.7
      | 317.15
      | 327.6
      | 338.05
      | 348.5
      | 358.95
      | 369.4
      | 379.85
      | 390.3
      | 400.75
      | 411.2
      | 421.65
      | 432.1
      | 442.55
      | 453
      | 463.45
      | 473.9
      | 484.35
      | 494.8
      | 505.25
      | 515.7
      | 526.15
      | 536.6
      | 547.05
      | 557.5
      | 567.95
      | 578.4
      | 588.85
      | 599.3
      | 609.75
      | 620.2
      | 630.65
      | 641.1
      | 651.55
      | 662
      | 672.45
      | 682.9
      | 693.35
      | 703.8
      | ]
  Add : Sum  Inputs=+-
  Add1 : Sum  Inputs=+-
  Constant1 : Constant  Value=10
  Constant2 : Constant  Value=4.8
  Constant3 : Constant  Value=0
  Constant4 : Constant  Value=5.8
  Divide : Product  Inputs=*/  OutDataTypeStr=double  RndMeth=Round
  Gain : Gain  Gain=0.9
  Logical Operator : Logic  AllPortsSameDT=off  OutDataTypeStr=boolean
  Relational Operator1 : RelationalOperator  Operator===  OutDataTypeStr=boolean  RndMeth=Simplest
  Relational Operator3 : RelationalOperator  OutDataTypeStr=boolean  RndMeth=Simplest
  Switch2 : Switch  Criteria=u2 ~= 0
  Ammonia_Slip : Outport
  Time : Outport  Port=2
  injector_On : Outport  Port=3
  wires:
  Pressure_sensor/1 -> Relational Operator1/1
  Add/1 -> [NOxIN_OUT]
  Constant1/1 -> Add/2
  Relational Operator1/1 -> Logical Operator/2
  Constant4/1 -> Relational Operator1/2
  NOx_Upstream/1 -> 1-D Lookup Table/1
  Constant2/1 -> Relational Operator3/2
  Relational Operator3/1 -> Logical Operator/1
  Constant3/1 -> Switch2/3
  Switch2/1 -> Divide/2
  Logical Operator/1 -> injector_On/1, Switch2/2
  [NOxIN_OUT] -> Add1/2
  Flow_Rate/1 -> Relational Operator3/1, Switch2/1
  Add1/1 -> Ammonia_Slip/1
  Gain/1 -> Divide/1, Add1/1
  Divide/1 -> Time/1
  1-D Lookup Table/1 -> Gain/1, Add/1

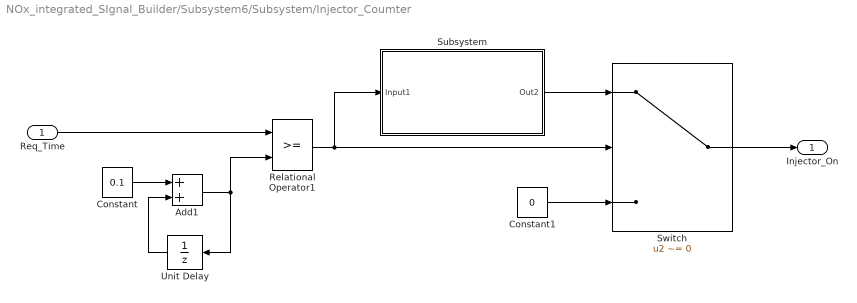
== system NOx_integrated_SIgnal_Builder/Subsystem6/Subsystem/Injector_Coumter ==
  Req_Time : Inport
  Add1 : Sum
  Constant : Constant  Value=0.1
  Constant1 : Constant  Value=0
  Relational Operator1 : RelationalOperator  OutDataTypeStr=boolean  RndMeth=Simplest
  Subsystem : Subsystem
  Switch : Switch  Criteria=u2 ~= 0
  Unit Delay : UnitDelay  SampleTime=-1  HasFrameUpgradeWarning=on
  Injector_On : Outport
  wires:
  Constant1/1 -> Switch/3
  Unit Delay/1 -> Add1/2
  Constant/1 -> Add1/1
  Add1/1 -> Unit Delay/1, Relational Operator1/2
  Subsystem/1(Out2) -> Switch/1
  Req_Time/1 -> Relational Operator1/1
  Switch/1 -> Injector_On/1
  Relational Operator1/1 -> Subsystem/1(Input1), Switch/2

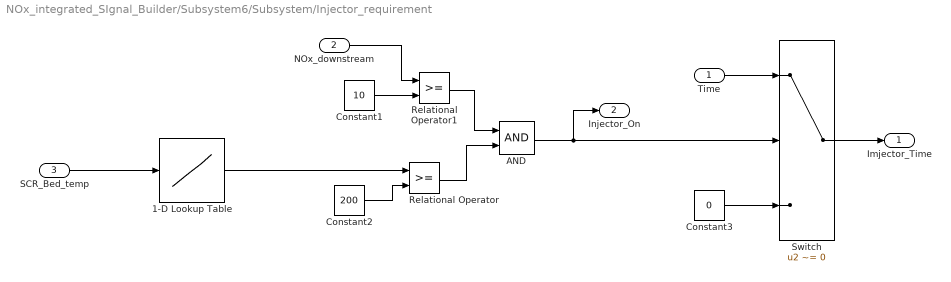
== system NOx_integrated_SIgnal_Builder/Subsystem6/Subsystem/Injector_requirement ==
  Time : Inport
  NOx_downstream : Inport  Port=2
  SCR_Bed_temp : Inport  Port=3
  1-D Lookup Table : Lookup_n-D  NumberOfTableDimensions=1  BreakpointsForDimension1=[1:10:650]  BreakpointsForDimension2=[1:1:500]  BreakpointsForDimension1DataTypeStr=double  Table=[1:10:650]  TableDataTypeStr=double  IntermediateResultsDataTypeStr=double  InternalRulePriority=Speed  OutDataTypeStr=double  RndMeth=Simplest  FractionDataTypeStr=double  InputSameDT=on
  AND : Logic  AllPortsSameDT=off  OutDataTypeStr=boolean
  Constant1 : Constant  Value=10
  Constant2 : Constant  Value=200
  Constant3 : Constant  Value=0
  Relational Operator : RelationalOperator  OutDataTypeStr=boolean  RndMeth=Simplest
  Relational Operator1 : RelationalOperator  OutDataTypeStr=boolean  RndMeth=Simplest
  Switch : Switch  Criteria=u2 ~= 0
  Imjector_Time : Outport
  Injector_On : Outport  Port=2
  wires:
  Constant1/1 -> Relational Operator1/2
  Constant2/1 -> Relational Operator/2
  Constant3/1 -> Switch/3
  1-D Lookup Table/1 -> Relational Operator/1
  AND/1 -> Injector_On/1, Switch/2
  Time/1 -> Switch/1
  Relational Operator1/1 -> AND/1
  Relational Operator/1 -> AND/2
  SCR_Bed_temp/1 -> 1-D Lookup Table/1
  Switch/1 -> Imjector_Time/1
  NOx_downstream/1 -> Relational Operator1/1

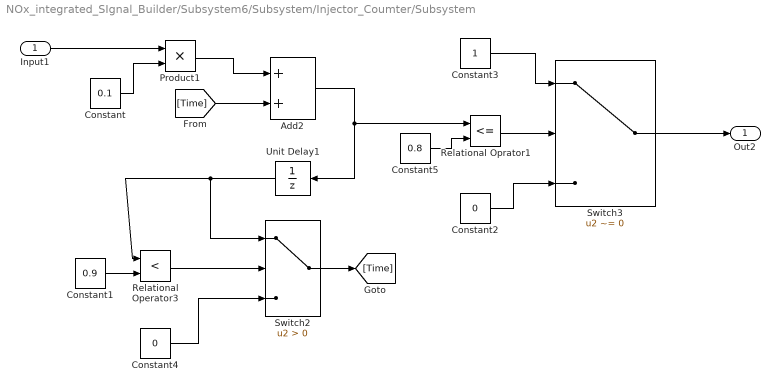
== system NOx_integrated_SIgnal_Builder/Subsystem6/Subsystem/Injector_Coumter/Subsystem ==
  Input1 : Inport
  Add2 : Sum
  Constant : Constant  Value=0.1
  Constant1 : Constant  Value=0.9
  Constant2 : Constant  Value=0
  Constant3 : Constant
  Constant4 : Constant  Value=0
  Constant5 : Constant  Value=0.8
  Product1 : Product
  Relational Operator3 : RelationalOperator  Operator=<  OutDataTypeStr=boolean  RndMeth=Simplest
  Relational Oprator1 : RelationalOperator  Operator=<=  OutDataTypeStr=boolean  RndMeth=Simplest
  Switch2 : Switch  Criteria=u2 > Threshold
  Switch3 : Switch  Criteria=u2 ~= 0
  Unit Delay1 : UnitDelay  SampleTime=-1  HasFrameUpgradeWarning=on
  Out2 : Outport
  wires:
  Unit Delay1/1 -> Relational Operator3/1, Switch2/1
  Relational Operator3/1 -> Switch2/2
  Constant3/1 -> Switch3/1
  Switch3/1 -> Out2/1
  Constant5/1 -> Relational Oprator1/2
  Constant/1 -> Product1/2
  Switch2/1 -> [Time]
  Product1/1 -> Add2/1
  Constant1/1 -> Relational Operator3/2
  Constant4/1 -> Switch2/3
  Input1/1 -> Product1/1
  Constant2/1 -> Switch3/3
  [Time] -> Add2/2
  Relational Oprator1/1 -> Switch3/2
  Add2/1 -> Relational Oprator1/1, Unit Delay1/1
